simulink model "System_Verification"  (R2021a)
settings: Solver=VariableStepAuto  StartTime=0.0  StopTime=20  RelTol=1e-3
libraries: simulink x1
settings Model: Creator=Lwando Kewute  LastModifiedBy=Lwando Kewute

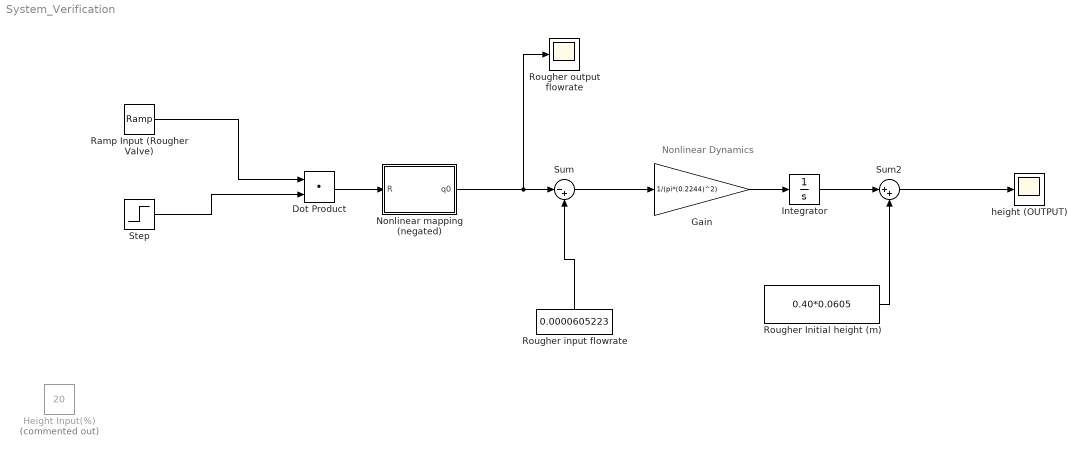
== system System_Verification ==
  note: Nonlinear Dynamics
  "     Rougher Initial height (m)" : Constant  Value=0.40*0.0605
  "   Rougher input flowrate" : Constant  Value=0.0000605223
  Dot Product : DotProduct  InputSameDT=on  OutDataTypeStr=Inherit: Inherit via internal rule
  Gain : Gain  Gain=1/(pi*(0.2244)^2)
  Height Input(%) : Constant  Commented=on  Value=20
  Integrator : Integrator
  Nonlinear mapping (negated) : MATLAB Function  TreatAsAtomicUnit=on
  Ramp Input (Rougher Valve) : simulink/Sources/Ramp  slope=-1  start=0  InitialOutput=10
  Rougher output flowrate : Scope
  Step : Step  Time=10  Before=1  After=0  SampleTime=0
  Sum : Sum  Inputs=|-+
  Sum2 : Sum  Inputs=|++
  height (OUTPUT) : Scope
  wires:
  Nonlinear mapping (negated)/1(q0) -> Rougher output flowrate/1, Sum/1
  Gain/1 -> Integrator/1
  Sum/1 -> Gain/1
  "   Rougher input flowrate"/1 -> Sum/2
  Ramp Input (Rougher Valve)/1 -> Dot Product/1
  Step/1 -> Dot Product/2
  Dot Product/1 -> Nonlinear mapping (negated)/1(R)
  Integrator/1 -> Sum2/1
  Sum2/1 -> height (OUTPUT)/1
  "     Rougher Initial height (m)"/1 -> Sum2/2

== matlab function System_Verification/Nonlinear mapping (negated) ==
  data: R input; q0 output
function q0 = fcn(R)

q0 = 5.7957623813336362e-005 * R^0 + -3.3937098753631659e-005 * R^1 + 1.8058143618083079e-005 * R^2 + -6.4199084190100935e-006 * R^3 +  1.1509077866801532e-006 * R^4 + -9.6876326648306145e-008 * R^5 + 3.0741104580358851e-009 * R^6;
%q0 = -q0;
